simulink model "simrfV2_powamp_dpd_comms"  (R2024b)
settings: Solver=FixedStepAuto  StartTime=0.0  StopTime=200e-2  RelTol=1e-3
PreLoadFcn:
  | BW =5e5;                       %  Signal BW
  | Tstep = 1/BW;                   %  Simulation BW BB
  | RF = 2.4e9;                       %  RF center frequency
  | IF = 50e6;                          % IF frequency
  | dataRatePA = 1/15.36e6;  % PA characterization sample time
  | M = 4;
  | FrameLength = 128;
  | 
  | load PAcoefficients;
undefined symbols (not defined in the file): rational, S, sparameters
libraries: simrfV2util1 x4, simrfV2elements x4, commrfcorlib x3, commrflib2 x2, commfilt2 x2, simrfV2_lib x2, dspstat3 x2, commrandsrc3 x1, commdigbbndam3 x1, dspmathops x1, simrfV2junction1 x1, simrfV2systems x1
Description:
  | Power Amplifier Characterization with DPD for Reduced Signal Distortion
settings Model: SimulationMode=accelerator  Creator=The MathWorks, Inc.  LastModifiedBy=93275
settings SolverCC: ZeroCrossAlgorithm=Adaptive  AlgebraicLoopSolver=TrustRegion
settings DataIOCC: LimitDataPoints=on  SaveFormat=Array  SaveOutput=off  SignalLogging=off  DSMLogging=off  SaveTime=off  ReturnWorkspaceOutputs=off
settings OptimizationCC: BlockReduction=off  BooleanDataType=off  LifeSpan=inf
settings DebuggingCC: SaveWithParameterizedLinksMsg=none  UnderspecifiedInitializationDetection=Classic  MergeDetectMultiDrivingBlocksExec=none  SignalResolutionControl=TryResolveAllWithWarning  UnconnectedInputMsg=warning  UnconnectedOutputMsg=warning  UnconnectedLineMsg=warning  AllowSymbolicDim=off  SFUnexpectedBacktrackingDiag=warning  SFNoUnconditionalDefaultTransitionDiag=warning  SFExecutionAtInitializationDiag=none  ArithmeticOperatorsInVariantConditions=warning
settings HardwareCC: ProdBitPerPointer=32  ProdBitPerSizeT=32  ProdBitPerPtrDiffT=32  ProdLargestAtomicFloat=None  ProdIntDivRoundTo=Undefined  ProdEndianess=Unspecified  ProdWordSize=32  ProdHWDeviceType=32-bit Generic  TargetBitPerPointer=64  TargetBitPerSizeT=64  TargetBitPerPtrDiffT=64  TargetLongLongMode=on  TargetIntDivRoundTo=Zero  TargetEndianess=LittleEndian  TargetWordSize=64  TargetHWDeviceType=MATLAB Host  ProdEqTarget=off
settings ModelReferenceCC: EnableRefExpFcnMdlSchedulingChecks=on  PropagateSignalLabelsOutOfModel=off
settings SFSimCC: SimUseLocalCustomCode=off  CustomCodeUndefinedFunction=UseInterfaceOnly
settings RTWCC: RTWUseLocalCustomCode=off  BuildConfiguration=Faster Runs  GPUComputeCapability=3.5
settings CodeAppCC: StateflowObjectComments=on
settings GRTTargetCC: TargetLangStandard=C89/C90 (ANSI)
settings ConfigComp: CovMetricSettings=dw  CovSaveCumulativeToWorkspaceVar=on  CovSaveSingleToWorkspaceVar=on  CovExternalEMLEnable=off
settings SimscapeCC: SimscapeNormalizeSystem=off

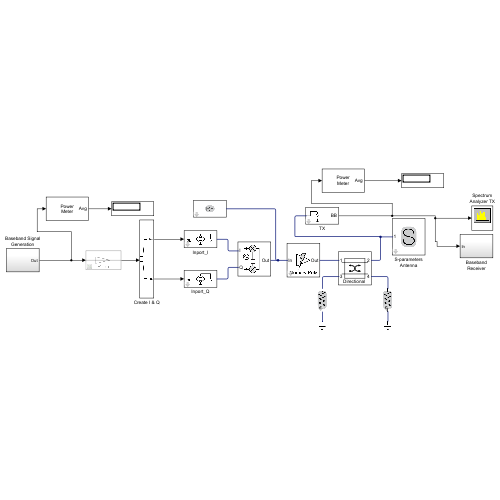
[thumbnail: Simulink's stored preview of the top-level diagram]
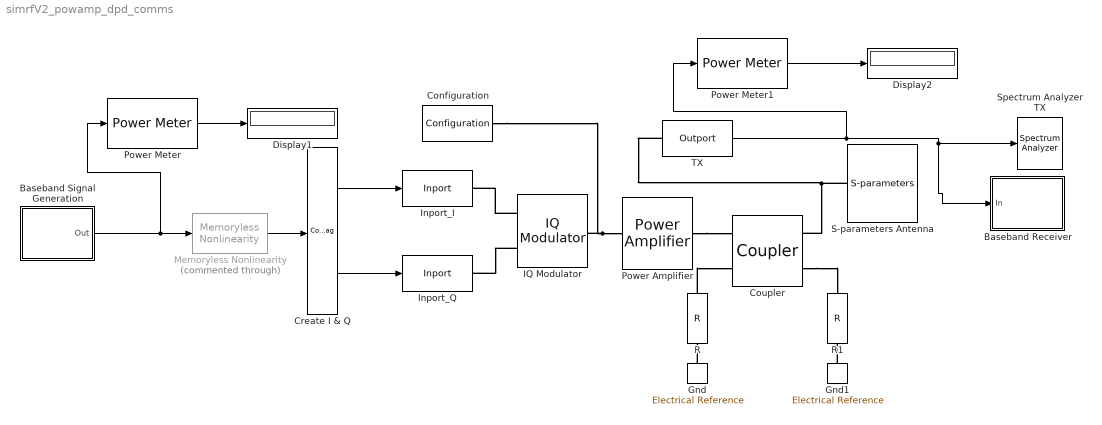
== system simrfV2_powamp_dpd_comms ==
  Baseband Receiver : Subsystem
  Baseband Signal Generation : Subsystem
  Configuration : simrfV2util1/Configuration  AutoFreq=off  Tones=[IF RF] Hz  Harmonics=[1 3]  NormalizeCarrierPower=on  SolverType=Auto  UseCCode=on  StepSize=Tstep s  AddNoise=on  defaultRNG=on  Seed=0  Temperature=290.0 K  SolverDelFlag=0  AbsTol=1e-6  RelTol=1e-3  MaxIter=10  ErrorEstimationType=2-norm over all variables  EnableInterpFilter=off  HiddenFIRfilterControllerParam=off  SmallSignalApprox=off  AllSimFreqs=on  SimFreqs=[] Hz  SimFreqsInternal=[]  SamplesPerFrame=FrameLength * M
  Coupler : simrfV2junction1/Coupler  classname=couplers  DataSource=Network-parameters  NumPorts=4  DeviceCirculator=Circulator clockwise  DeviceDivider=T power divider  DeviceCoupler=Directional coupler  Paramtype=S-parameters  Sparam=[0 0 1; 1 0 0; 0 1 0]  SparamFreq=1e9 Hz  SparamZ0=50  Phase12=0  Phase33=0  Alpha=0  NumberDividerOutports=2  Coupling=50  Directivity=22  InsertionLoss=0.3  ReturnLoss=35  InternalGrounding=on  SparamRepresentation=Frequency domain  FitOpt=Share all poles  FitTol=-40  MaxPoles=48
  Create I & Q : ComplexToRealImag
  Display1 : Display
  Display2 : Display
  Gnd : simrfV2_lib/Elements/Electrical Reference
      settings: InternalSimscapePortConfiguration="{\"Bottom\":[],\"Left\":[{\"id\":\"V\",\"label\":\"\",\"type\":\"foundation.rf.circuitenvelope\"}],\"Right\":[],\"Top\":[]}"
  Gnd1 : simrfV2_lib/Elements/Electrical Reference
      settings: InternalSimscapePortConfiguration="{\"Bottom\":[],\"Left\":[{\"id\":\"V\",\"label\":\"\",\"type\":\"foundation.rf.circuitenvelope\"}],\"Right\":[],\"Top\":[]}"
  IQ Modulator : simrfV2systems/IQ Modulator  classname=iqmod  Source_linear_gain=Available power gain  linear_gain=0 dB  Poly_Coeffs=[0 1]  LOFreq=RF Hz  Zin=50  Zout=50  AddIRFilters=off  AddCSFilter=on  InternalGrounding=on  ForceNextInit=off  NFloor=-168  GainMismatch=-0.25 dB  PhaseMismatch=0.06 deg  Isolation=inf dB  AddPhaseNoise=off  PhaseNoiseOffset=1e6  PhaseNoiseLevel=-140  AutoImpulseLengthPN=on  ImpulseLengthPN=1e-10  ImpulseLength_unitPN=s  Source_Poly=Even and odd order  IPType=Input  IP2=inf dBm  IP3=inf dBm  P1dB=inf dBm  Psat=inf dBm  Gcomp=inf dBm  DesignMethodIR=Ideal  ResponseTypeIR=Lowpass  ImplementationIR=LC Tee  ImplementationIdealIR=Constant per carrier  ImplementationRationalIR=Transfer function  UseFilterOrderIR=on  FilterOrderIR=3  PassFreq_lpIR=1  PassFreq_lp_unitIR=GHz  PassFreq_hpIR=2  PassFreq_hp_unitIR=GHz  PassFreq_bpIR=[2 3]  PassFreq_bp_unitIR=GHz  PassFreq_bsIR=[1 4]  PassFreq_bs_unitIR=GHz  PassAttenIR=10*log10(2)  StopFreq_lpIR=2  StopFreq_lp_unitIR=GHz  StopFreq_hpIR=1  StopFreq_hp_unitIR=GHz  StopFreq_bpIR=[1.5 3.5]  StopFreq_bp_unitIR=GHz  StopFreq_bsIR=[2.1 2.9]  StopFreq_bs_unitIR=GHz  StopAttenIR=40  RsrcIR=50  RloadIR=50  AutoImpulseLengthIR=on  ImpulseLengthIR=1e-10  ImpulseLength_unitIR=s  DesignMethodCS=Ideal  ResponseTypeCS=Highpass  ImplementationCS=LC Tee  ImplementationIdealCS=Constant per carrier  ImplementationRationalCS=Transfer function  UseFilterOrderCS=on  FilterOrderCS=3  PassFreq_lpCS=1  PassFreq_lp_unitCS=GHz  PassFreq_hpCS=2  PassFreq_hp_unitCS=GHz  PassFreq_bpCS=[2 3]  PassFreq_bp_unitCS=GHz  PassFreq_bsCS=[1 4]  PassFreq_bs_unitCS=GHz  PassAttenCS=10*log10(2)  StopFreq_lpCS=2  StopFreq_lp_unitCS=GHz  StopFreq_hpCS=1  StopFreq_hp_unitCS=GHz  StopFreq_bpCS=[1.5 3.5]  StopFreq_bp_unitCS=GHz  StopFreq_bsCS=[2.1 2.9]  StopFreq_bs_unitCS=GHz  StopAttenCS=40  RsrcCS=50  RloadCS=50  AutoImpulseLengthCS=on  ImpulseLengthCS=1e-10  ImpulseLength_unitCS=s
  Inport_I : simrfV2util1/Inport  SimulinkInputSignalType=Ideal voltage  CarrierFreq=0 Hz  ZS=0  UseSqWave=off  NumCoeff=10  Bias=0  DutyCyc=50  InternalGrounding=on
  Inport_Q : simrfV2util1/Inport  SimulinkInputSignalType=Ideal voltage  CarrierFreq=0 Hz  ZS=0  UseSqWave=off  NumCoeff=10  Bias=0  DutyCyc=50  InternalGrounding=on
  Memoryless Nonlinearity : commrflib2/Memoryless Nonlinearity  Commented=through  Model=modified-rapp  Gain=0  Nonlinearity=IIP3  IIP3=45  OIP3=Inf  IP1dB=Inf  OP1dB=Inf  IPsat=Inf  OPsat=Inf  Table=[ -25, 5, -1; -10, 20, -2; 0, 27, 5; 5, 28, 12 ]  MagnitudeGainDB=7.5  Vsat=6.5  MagnitudeSmooth=3.5  PhaseGainRadian=-.45  PhaseSaturation=.88  PhaseSmooth=3.43  InputScaleDB=0  AmAmParameters=[6.6492, 0.8832]  AmPmParameters=[0.1528, 0.5296]  OutputScaleDB=0  ReferenceLoad=1  SimulateUsing=Code generation
  Power Amplifier : simrfV2elements/Power Amplifier  classname=poweramp  ModelType=Memory polynomial  CoeffMatrix=[1 0 -0.5827-0.0096i 0 0.0537+0.0029i]  UnitDelay=1e-6  Rin=50  Rout=50  InternalGrounding=on
  Power Meter : dspstat3/Power Meter  Measurement=Average power  ReferenceLoad=1  OutputPowerUnits=dBm  WindowLength=256  OverlapLength=255  AllowArbitraryInputLength=on  ComputeCCDF=off  PowerRange=50  PowerResolution=0.1  CCDFOutput=Relative power (dB above average power)  ProbabilityVector=[ 10; 1; 0.1; 0.01; 0.001; 0.0001 ]  RelativePowerVector=[ 0; 3; 6; 9; 12 ]  ResetPort=off  SimulateUsing=Code generation
      settings: LibrarySourceBlock=commutil2/Power Meter
  Power Meter1 : dspstat3/Power Meter  Measurement=Average power  ReferenceLoad=1  OutputPowerUnits=dBm  WindowLength=256  OverlapLength=255  AllowArbitraryInputLength=on  ComputeCCDF=off  PowerRange=50  PowerResolution=0.1  CCDFOutput=Relative power (dB above average power)  ProbabilityVector=[ 10; 1; 0.1; 0.01; 0.001; 0.0001 ]  RelativePowerVector=[ 0; 3; 6; 9; 12 ]  ResetPort=off  SimulateUsing=Code generation
      settings: LibrarySourceBlock=commutil2/Power Meter
  R : simrfV2elements/R  classname=resistor  Resistance=50 Ohm  AddNoise=on
  R1 : simrfV2elements/R  classname=resistor  Resistance=50 Ohm  AddNoise=on
  S-parameters Antenna : simrfV2elements/S-parameters  classname=sparam_element  DataSource=Data file  File=antenna.s1p  isNetworkObj=off  NetworkObject=sparameters('default.s2p')  Paramtype=S-parameters  Sparam=[0 0;1 0]  SparamFreq=1e9 Hz  SparamZ0=50  isRationalObj=off  RationalObject=rational('default.s2p')  Residues=0  Poles=0  DF={0 0; 1 0}  FitOpt=Fit individually  FitTol=-40  MaxPoles=48  SourceFreq=Extracted from data source  PlotFreq=[1e9:1e6:3e9] Hz  PlotType=X-Y plane  YParam1=S(1,1)  YFormat1=Magnitude (dB)  YParam2=None  YFormat2=Magnitude (dB)  YOption=Linear  XOption=Linear  AddNoise=on  InternalGrounding=on  SparamRepresentation=Frequency domain  AutoImpulseLength=on  ImpulseLength=1e-10 s  MagModeling=off  CacheLevel=0
  Spectrum Analyzer TX : SpectrumAnalyzer  WindowPosition=[627.000000,180.000000,1093.000000,626.000000,]  ScopeFrameLocation=window  Method=Welch  SampleRate=50000000  AxesScaling=Manual  Span=1843200000  StartFrequency=-921600000  StopFrequency=921600000  AveragingMethod=Running  SpectralAverages=6  ReferenceLoad=50  YLimits=[-51.12191047508542141,3.8675431920021758891]  AllowFFTLengthLessThanSamplesPerUpdate=on  DefaultConfigurationName=spbscopes.SpectrumAnalyzerBlockCfg  IsFrequencyInputMode=0  FrequencyVectorPort=0  FrequencyVectorFromPort=0  FrequencyInputRBWPort=0  FrequencyInputRBWFromPort=0
  TX : simrfV2util1/Outport  SensorType=Ideal voltage  OutputFormat=Complex Baseband  CarrierFreq=RF Hz  ZL=Inf  InternalGrounding=on  StepSize=-1 s  AutoStep=off  HalfPolyphaseLength=0
  wires:
  Create I & Q/2 -> Inport_Q/1
  Create I & Q/1 -> Inport_I/1
  Baseband Signal Generation/1(Out) -> Power Meter/1, Memoryless Nonlinearity/1
  Power Meter/1 -> Display1/1
  Power Meter1/1 -> Display2/1
  TX/1 -> Power Meter1/1, Baseband Receiver/1(In), Spectrum Analyzer TX/1
  Memoryless Nonlinearity/1 -> Create I & Q/1
  connections:
  IQ Modulator/LConn1 -- Inport_I/RConn1
  IQ Modulator/LConn2 -- Inport_Q/RConn1
  R/LConn1 -- Coupler/LConn2
  Gnd/LConn1 -- R/RConn1
  S-parameters Antenna/LConn1 -- TX/LConn1 -- Coupler/RConn1
  Gnd1/LConn1 -- R1/RConn1
  Coupler/RConn2 -- R1/LConn1
  Configuration/LConn1 -- Power Amplifier/LConn1 -- IQ Modulator/RConn1
  Power Amplifier/RConn1 -- Coupler/LConn1

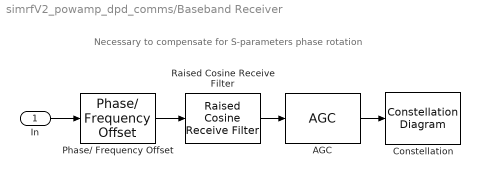
== system simrfV2_powamp_dpd_comms/Baseband Receiver ==
  note: Necessary to compensate for S-parameters phase rotation
  In : Inport
  AGC : commrfcorlib/AGC  LegacyMode=off  DetectorMethod=Rectifier  LoopMethod=Linear  UpdatePeriod=100  StepSize=0.1  AdaptationStepSize=0.01  DesiredOutputPower=1  AveragingLength=FrameLength  MaximumGain=30  MaxPowerGain=100  GainOutputPort=off  InputPowerOutputPort=off  SimulateUsing=Interpreted execution
  Constellation : ConstellationDiagram  Tag=ScatterPlot  WindowPosition=[137.000000,263.000000,647.000000,543.000000,]  ScopeFrameLocation=window  SymbolsToDisplaySource=Property  SymbolsToDisplay=512  ReferenceConstellation="[-0.94868+0.94868i        -0.94868+0.31623i        -0.94868-0.31623i        -0.94868-0.94868i        -0.31623+0.94868i        -0.31623+0.31623i        -0.31623-0.31623i        -0.31623-0.94868i         0.31623+0.94868i         0.31623+0.31623i         0.31623-0.31623i         0.31623-0.94868i         0.94868+0.94868i         0.94868+0.31623i         0.94868-0.31623i         0.94868-0.94868i]"  Title=RX signal constellation  XLimits=[-1.4,1.35]  YLimits=[-1.77,1.72]  ColorFading=on  EnableMeasurements=on  MeasurementInterval=512  DefaultConfigurationName=comm.scopes.ConstellationDiagramBlockCfg
  Phase/ Frequency Offset : commrflib2/Phase// Frequency Offset  phaseOffset=0  freqPort=off  freqOffset=0
  Raised Cosine Receive Filter : commfilt2/Raised Cosine Receive Filter  filtType=Square root  R=0.2  filtSpan=10  N=M  downFactor=M  downOffset=0  filterGain=1  InputProcessing=Columns as channels (frame based)  RateOptions=Enforce single-rate processing  framing=Mute  checkCoeff=off  variableName=rcRxFilt1  currentFiltSpan=10  D=(10)/2  inputOffset=0  sampMode=Mute  saveAsFlag=0  rateMode=Downsampling  checkGain=Normalized  launchFVT=on  roundingMode=Floor  overflowMode=off  coeffDataTypeStr=Inherit: Same word length as input  coeffMin=[]  coeffMax=[]  coeffLastDataTypeStr=Inherit: Same word length as input  accumDataTypeStr=Inherit: Same as product output  accumLastDataTypeStr=Inherit: Same as product output  outputDataTypeStr=Inherit: Same as accumulator  outputMin=[]  outputMax=[]  outputLastDataTypeStr=Inherit: Same as accumulator
  wires:
  Raised Cosine Receive Filter/1 -> AGC/1
  In/1 -> Phase/ Frequency Offset/1
  Phase/ Frequency Offset/1 -> Raised Cosine Receive Filter/1
  AGC/1 -> Constellation/1

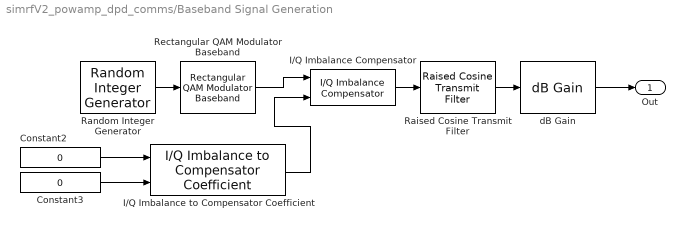
== system simrfV2_powamp_dpd_comms/Baseband Signal Generation ==
  Constant2 : Constant  Value=0
  Constant3 : Constant  Value=0
  I/Q Imbalance Compensator : commrfcorlib/I//Q Imbalance Compensator  CoefficientSource=Input port  InitialCoefficient=0 + 0j  StepSizeSource=Property  StepSize=0.00001  AdaptInputPort=off  CoefficientOutputPort=off  SimulateUsing=Code generation
  I/Q Imbalance to Compensator Coefficient : commrfcorlib/I//Q Imbalance to Compensator Coefficient
  Raised Cosine Transmit Filter : commfilt2/Raised Cosine Transmit Filter  filtType=Square root  R=0.2  filtSpan=10  N=M  filterGain=1  InputProcessing=Columns as channels (frame based)  RateOptions=Enforce single-rate processing  framing=Mute  checkCoeff=off  variableName=rcTxFilt1  checkGain=Normalized  sampMode=Mute  saveAsFlag=0  currentFiltSpan=10  D=(10)/2  launchFVT=on  roundingMode=Floor  overflowMode=off  coeffDataTypeStr=Inherit: Same word length as input  coeffMin=[]  coeffMax=[]  coeffLastDataTypeStr=Inherit: Same word length as input  outputDataTypeStr=Inherit: Same as accumulator  outputMin=[]  outputMax=[]  outputLastDataTypeStr=Inherit: Same as accumulator
  Random Integer Generator : commrandsrc3/Random Integer Generator  SetSize=2^M  SeedSource=Parameter  Seed=37  SampleTime=Tstep*M  SamplesPerFrame=FrameLength  OutputDataType=double  SimulateUsing=Interpreted execution
  Rectangular QAM Modulator Baseband : commdigbbndam3/Rectangular QAM Modulator Baseband  M=2^M  InType=Integer  Enc=Gray  Mapping=[0:15]  PowType=Average Power  MinDist=2  AvgPow=1  PeakPow=1  Ph=0  outDtype=double  outWordLen=16  outUDDataType=sfix(16)  outFracLenMode=Best precision  outFracLen=15  outDataTypeStr=double  outLastDataTypeStr=double
  dB Gain : dspmathops/dB Gain  dB=0  intype=Amplitude
  Out : Outport  VectorParamsAs1DForOutWhenUnconnected=off
  wires:
  Random Integer Generator/1 -> Rectangular QAM Modulator Baseband/1
  Raised Cosine Transmit Filter/1 -> dB Gain/1
  Constant3/1 -> I/Q Imbalance to Compensator Coefficient/2
  Constant2/1 -> I/Q Imbalance to Compensator Coefficient/1
  Rectangular QAM Modulator Baseband/1 -> I/Q Imbalance Compensator/1
  I/Q Imbalance to Compensator Coefficient/1 -> I/Q Imbalance Compensator/2
  dB Gain/1 -> Out/1
  I/Q Imbalance Compensator/1 -> Raised Cosine Transmit Filter/1
